simulink model "BESS_grid_test"  (Simulink 8.1)
settings: Solver=ode1  StartTime=0.0  StopTime=inf  FixedStep=Ts  MaxStep=1e-3  RelTol=1e-3
PostLoadFcn:
  | NREL_Mode=3; BANSHEE_init; init_EssTest;
InitFcn:
  | NREL_Mode=3; BANSHEE_init; init_EssTest;
values from neighbouring files (symbols this model uses):
  DER_REL = xlsread('DER_relay.xlsx')    [relay_settings_init.m]
  Ts = 100E-6    (= 0.0001)    [BANSHEE_init.m]    (also in Ghost_init.m)
undefined symbols (not defined in the file or in its folder): CBID, Stim
libraries: simulink x31, breaker_lib x3, rtlab x2, transformer_lib x2, artemis x1, cables_lib x1, BESS_lib x1, relay_modbus_lib x1, rtio_generic_modbus x1, rtio_opalrt_ml605ex1 x1, TestSeq_slave_lib x1, controllable_grid_lib x1
settings Model: ARTEMISmethode_block_infos=$$__separator__$$BESS_grid_test/ARTEMIS Guide$$__separator__$$  Creator=RE25624  LastModifiedBy=pkoralew  BufferReuse=off
settings SolverCC: ZeroCrossAlgorithm=Adaptive
settings DataIOCC: ExternalInput=getinputstruct(op_snapshot1)  InitialState=getstatestruct(op_snapshot1)  LimitDataPoints=off  MaxDataPoints=90060  SignalLoggingSaveFormat=Dataset  SaveOutput=off  SignalLogging=off  DSMLogging=off  SaveTime=off  OutputSaveName=result
settings OptimizationCC: BlockReduction=off  OptimizeBlockIOStorage=off  BufferReuse=off  ExpressionFolding=off  LocalBlockOutputs=off
settings DebuggingCC: MaxConsecutiveZCsMsg=warning  IgnoredZcDiagnostic=none  SolverPrmCheckMsg=none  MultiTaskRateTransMsg=warning  ParameterPrecisionLossMsg=none  FcnCallInpInsideContextMsg=EnableAllAsWarning  FrameProcessingCompatibilityMsg=error  ModelReferenceExtraNoncontSigs=warning
settings ModelReferenceCC: UpdateModelReferenceTargets=IfOutOfDate
settings SFSimCC: SFSimEcho=off
settings GRTTargetCC: CodeReplacementLibrary=C89/C90 (ANSI)

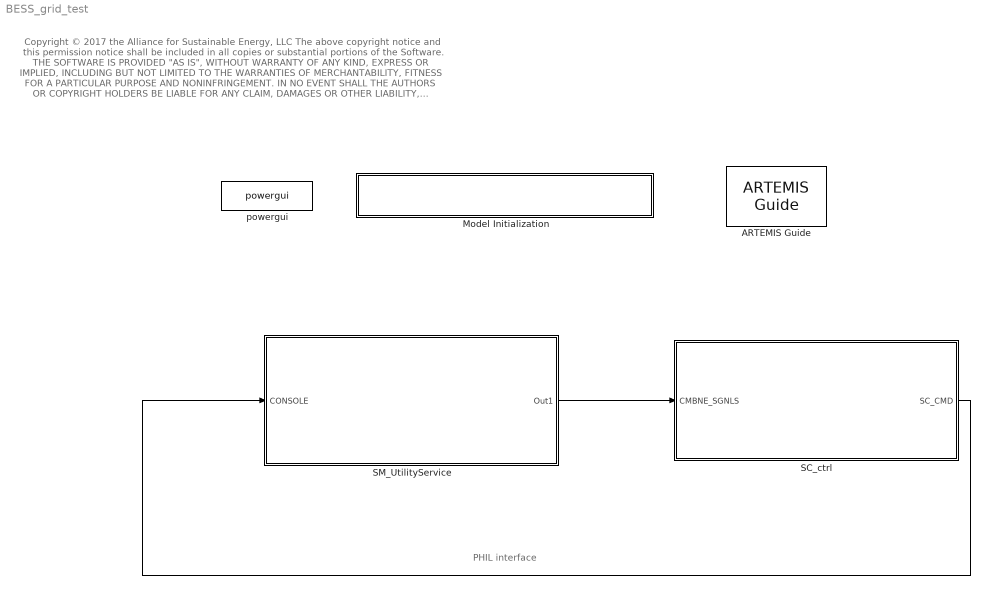
== system BESS_grid_test ==
  note: PHIL interface
  note: Copyright © 2017 the Alliance for Sustainable Energy, LLC
      |
      | The above copyright notice and this permission notice shall be included in all copies or substantial portions of the Software.
      |
      | THE SOFTWARE IS PROVIDED "AS IS", WITHOUT WARRANTY OF ANY KIND, EXPRESS OR IMPLIED, INCLUDING
      | BUT NOT LIMITED TO THE WARRANTIES OF MERCHANTABILITY, FITNESS FOR A PARTICULAR PURPOSE AND
      | NONINFRINGEMENT. IN NO EVENT SHALL THE AUTHORS OR COPYRIGHT HOLDERS BE LIABLE FOR ANY CLAIM,
      |  DAMAGES OR OTHER LIABILITY, WHETHER IN AN ACTION OF CONTRACT, TORT OR OTHERWISE, ARISING FROM,
      | OUT OF OR IN CONNECTION WITH THE SOFTWARE OR THE USE OR OTHER DEALINGS IN THE SOFTWARE
  ARTEMIS Guide : artemis/ARTEMIS/ARTEMIS Guide  Tag=FTSSmethode_opal_4hx0r99  Description=5.0_z1  lock=on  Ts=Ts  opt=art5  dyna=off  nb_perm=4  RT_fullcomp=off  ssn=on  ssn_itvc=off  ssn_ivic=off  ssn_ext=off  ssn_solver=Art5 with Backward Euler nodal interface  ssn_impulse=off  ssn_quasimpulse=off  ssn_impulse_loop=5  paraExtinctionThy=off  Thy_Impulse=on  dtc=Off  dtc_opt=normal  ao=on  simtype=off  ct_mac=off  lin_mov=off  lsp=[0.001 2]  spike_skip=Disabled  dtc_extra=1  dtc_sws=normal  dtc_pied=0.5  SPSRulesBlock=SPSRules  tre=on  ctmm=off  LF=off  dpl_type=ARTEMiS DPL  rlc_type=off  custom_type=off  para=on  ssn_ImpulseLoopBlockedStateUpdate=5  ssn_mov_iter_number=5  ssn_switch_iter_number=5  ssn_nib_type_verify=on
  Model Initialization : Subsystem  AncestorBlock=artemis/Tools /Misc/Model Initialization  mask(Model Functions){InitFcnX=NREL_Mode=3; BANSHEE_init; init_EssTest;, prel=off, posl=on, inif=on, strf=off}
      mask prompts: InitFcnX "Initialisation"; prel "Preload Function"; posl "PostLoad Function"; inif "InitFcn"; strf "StartFcn"
      mask init:
      | currentBlock = gcb;
      | root = bdroot(currentBlock);
      | 
      | if ~strcmp(get_param(root,'BlockDiagramType'),'library')
      |     if prel==1
      |         set_param(root, 'PreLoadFcn', InitFcnX);
      |     else
      |         set_param(root, 'PreLoadFcn', '');
      |     end
      |     if inif==1
      |         set_param(root, 'InitFcn', InitFcnX);
      |     else
      |         set_param(root, 'InitFcn', '');
      |     end
      |     if strf==1
      |         set_param(root, 'StartFcn', InitFcnX);
      |     else
      |         set_param(root, 'StartFcn', '');
      |     end
      |     if posl==1
      |         set_param(root, 'PostLoadFcn', InitFcnX);
      |     else
      |         set_param(root, 'PostLoadFcn', '');
      |     end
      | end
      | 
      | pos = get_param(currentBlock, 'Position');
      | width = pos(3) - pos(1); height = pos(4) - pos(2);
      | txt = [ upper(root) '\n' '- InitFcn. . . . . '  get_param(root, 'InitFcn') ];
      settings: CopyFcn=set_param(gcb,'LinkStatus','inactive')
      mask Display: text(5, height*0.5, txt, 'horizontalAlignment', 'left', 'verticalAlignment', 'middle') ;
  SC_ctrl : Subsystem
  SM_UtilityService : Subsystem
  powergui : powerlib/powergui  Priority=2  SimulationMode=Discrete  SolverType=Tustin  SampleTime=Ts  frequency=60  SPID=off  DisableSnubberDevices=off  DisableRonSwitches=off  DisableVfSwitches=off  SwTol=0  Interpol=off  DisplayEquations=off  frequencyindice=0  Pbase=100e6  ErrMax=1e-4  Iterations=50  UnitsV=kV  UnitsW=MW  FunctionMessages=off  echomessages=off  HookPort=off  EnableUseOfTLC=off  x0status=blocks  RestoreLinks=warning  ResistiveCurrentMeasurement=off  Frange=logspace(0,3,50)  Ylog=off  Xlog=off  ShowGrid=off  save=off  variable=ZData  structure=0  ZoomFFT=on  StartTime=0.0  cycles=2  DisplayStyle=off  fundamental=60  FreqAxis=off  MaxFrequency=1000  frequencyindicesteady=1  RmsSteady=1  display=off  Ts=0  methode=off
  wires:
  SC_ctrl/1(SC_CMD) -> SM_UtilityService/1(CONSOLE)
  SM_UtilityService/1(Out1) -> SC_ctrl/1(CMBNE_SGNLS)

== system BESS_grid_test/Model Initialization ==

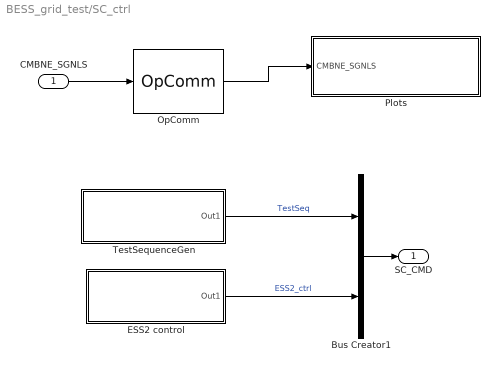
== system BESS_grid_test/SC_ctrl ==
  CMBNE_SGNLS : Inport
  Bus Creator1 : BusCreator  Inputs=2
  ESS2 control : Subsystem
  OpComm : rtlab/OpComm  nbport=1  groupe_acq=1  subsys_rate=0  st=0  Synchronization=on  Interpolation=on  Threshold=1.0  Missed_Data=off  Sim_Time=off  Samples=off  dynSigOut=off  from_console=0  warning_done=off  writeOpCommFile=off  Offset=off
  Plots : Subsystem
  TestSequenceGen : Subsystem
  SC_CMD : Outport
  wires:
  CMBNE_SGNLS/1 -> OpComm/1
  Bus Creator1/1 -> SC_CMD/1
  ESS2 control/1(Out1) -> Bus Creator1/2  "ESS2_ctrl"
  OpComm/1 -> Plots/1(CMBNE_SGNLS)
  TestSequenceGen/1(Out1) -> Bus Creator1/1  "TestSeq"

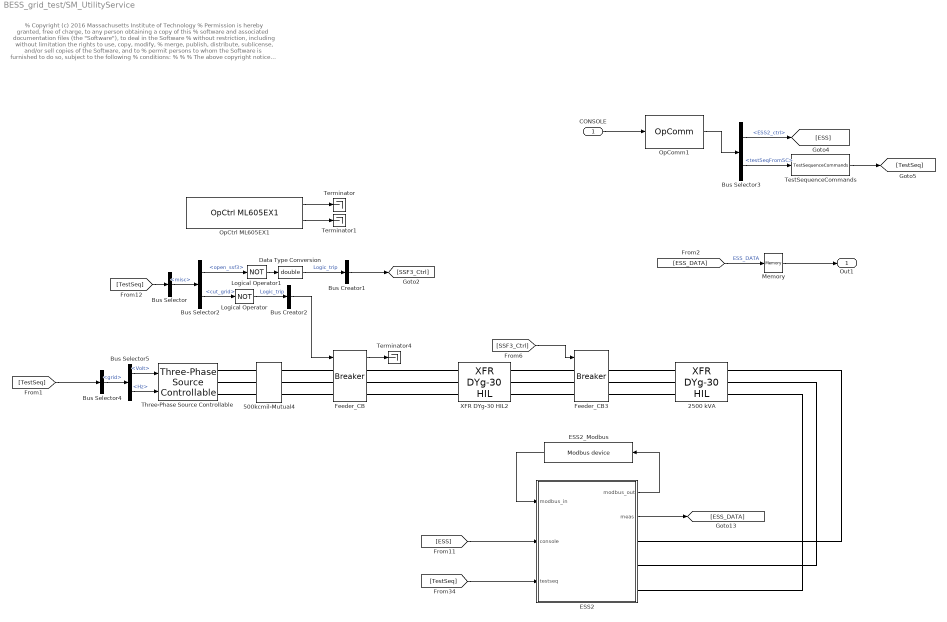
== system BESS_grid_test/SM_UtilityService ==
  note: % Copyright (c) 2016 Massachusetts Institute of Technology
      | % Permission is hereby granted, free of charge, to any person obtaining a copy of this
      | % software and associated documentation files (the "Software"), to deal in the Software
      | % without restriction, including without limitation the rights to use, copy, modify,
      | % merge, publish, distribute, sublicense, and/or sell copies of the Software, and to
      | % permit persons to whom the Software is furnished to do so, subject to the following
      | % conditions:
      | %
      | %
      | % The above copyright notice and this permission notice shall be included in
      | % all copies or substantial portions of the Software.
      | %
      | % THE SOFTWARE IS PROVIDED "AS IS", WITHOUT WARRANTY OF ANY KIND, EXPRESS OR IMPLIED,
      | % INCLUDING BUT NOT LIMITED TO THE WARRANTIES OF MERCHANTABILITY, FITNESS FOR A
      | % PARTICULAR PURPOSE AND NONINFRINGEMENT. IN NO EVENT SHALL THE AUTHORS OR COPYRIGHT
      | % HOLDERS BE LIABLE FOR ANY CLAIM, DAMAGES OR OTHER LIABILITY, WHETHER IN AN ACTION
      | % OF CONTRACT, TORT OR OTHERWISE, ARISING FROM, OUT OF OR IN CONNECTION WITH THE
      | % SOFTWARE OR THE USE OR OTHER DEALINGS IN THE SOFTWARE.
      | %
      | %
      | %%
  CONSOLE : Inport
  2500 kVA : transformer_lib/XFR DYg-30 HIL  Rating=2500  Vp=13800  Vs=480  Z=5.56  XR=5.52
  500kcmil-Mutual4 : cables_lib/500kcmil-Mutual  length=50  par_sets=1  ratio=3
  Bus Creator1 : BusCreator  Inputs=1
  Bus Creator2 : BusCreator  Inputs=1
  Bus Selector : BusSelector  OutputSignals=misc
  Bus Selector2 : BusSelector  OutputSignals=open_ssf3,cut_grid
  Bus Selector3 : BusSelector  OutputSignals=ESS2_ctrl,TestSeq.testSeqFromSC
  Bus Selector4 : BusSelector  OutputSignals=grid
  Bus Selector5 : BusSelector  OutputSignals=Volt,Hz
  Data Type Conversion : DataTypeConversion  OutDataTypeStr=double
  ESS2 : Subsystem
  ESS2_Modbus : rtio_generic_modbus/Modbus device  conf_name=ESS2_modbus.opal  conf_name_mask=ESS2_modbus.xls  sample_time=Ts
  Feeder_CB : breaker_lib/Breaker  Ts=Ts  mech_delay=cb_mech_delay
  Feeder_CB3 : breaker_lib/Breaker  Ts=Ts  mech_delay=cb_mech_delay
  Logical Operator : Logic  Operator=NOT  AllPortsSameDT=off  OutDataTypeStr=boolean
  Logical Operator1 : Logic  Operator=NOT  AllPortsSameDT=off  OutDataTypeStr=boolean
  Memory : Memory
  OpComm1 : rtlab/OpComm  nbport=1  groupe_acq=1  subsys_rate=0  st=0  Synchronization=on  Interpolation=on  Threshold=1.0  Missed_Data=off  Sim_Time=off  Samples=off  dynSigOut=off  from_console=1  warning_done=off  writeOpCommFile=off  Offset=off
  OpCtrl ML605EX1 : rtio_opalrt_ml605ex1/OpCtrl ML605EX1  CtrlName='ML605EX1 Ctrl'  boardid=4  BitstreamFilename=ML605_2-EX-0029-2_2_4_33-32AIO_16DIO16SelectableDIO-10-01.bin  numconfig=-1  mode=Master  externalClock=off  decimRtsi=0  calibIO=off  SampleTime=0  loadinport=-1
  Terminator : Terminator
  Terminator1 : Terminator
  Terminator4 : Terminator
  TestSequenceCommands : TestSeq_slave_lib/TestSequenceCommands
  Three-Phase Source Controllable : controllable_grid_lib/Three-Phase Source Controllable  Ts=Ts  Rg=0.8  Lg=16.58e-3
  XFR DYg-30 HIL2 : transformer_lib/XFR DYg-30 HIL  Rating=50000  Vp=115000  Vs=13800  Z=6  XR=30
  Out1 : Outport
  wires:
  CONSOLE/1 -> OpComm1/1
  OpComm1/1 -> Bus Selector3/1
  Feeder_CB/1 -> Terminator4/1
  [TestSeq] -> Bus Selector/1
  Logical Operator/1 -> Bus Creator2/1  "Logic_trip"
  Bus Creator2/1 -> Feeder_CB/1
  [SSF3_Ctrl] -> Feeder_CB3/1
  OpCtrl ML605EX1/1 -> Terminator/1
  OpCtrl ML605EX1/2 -> Terminator1/1
  Bus Selector/1 -> Bus Selector2/1  "<misc>"
  Bus Selector2/2 -> Logical Operator/1  "<cut_grid>"
  Bus Selector2/1 -> Logical Operator1/1  "<open_ssf3>"
  Logical Operator1/1 -> Data Type Conversion/1
  Bus Creator1/1 -> [SSF3_Ctrl]
  Data Type Conversion/1 -> Bus Creator1/1  "Logic_trip"
  [TestSeq] -> Bus Selector4/1
  Bus Selector4/1 -> Bus Selector5/1  "<grid>"
  Bus Selector5/2 -> Three-Phase Source Controllable/2  "<Hz>"
  Bus Selector5/1 -> Three-Phase Source Controllable/1  "<Volt>"
  [ESS] -> ESS2/2(console)
  ESS2/2(meas) -> [ESS_DATA]
  ESS2/1(modbus_out) -> ESS2_Modbus/1
  ESS2_Modbus/1 -> ESS2/1(modbus_in)
  [TestSeq] -> ESS2/3(testseq)
  [ESS_DATA] -> Memory/1  "ESS_DATA"
  Memory/1 -> Out1/1
  Bus Selector3/1 -> [ESS]  "<ESS2_ctrl>"
  Bus Selector3/2 -> TestSequenceCommands/1  "<testSeqFromSC>"
  TestSequenceCommands/1 -> [TestSeq]
  connections:
  500kcmil-Mutual4/RConn3 -- Feeder_CB/LConn3
  500kcmil-Mutual4/RConn2 -- Feeder_CB/LConn2
  500kcmil-Mutual4/RConn1 -- Feeder_CB/LConn1
  Three-Phase Source Controllable/RConn3 -- 500kcmil-Mutual4/LConn3
  Three-Phase Source Controllable/RConn1 -- 500kcmil-Mutual4/LConn1
  Three-Phase Source Controllable/RConn2 -- 500kcmil-Mutual4/LConn2
  2500 kVA/RConn2 -- ESS2/RConn2
  2500 kVA/RConn1 -- ESS2/RConn1
  2500 kVA/RConn3 -- ESS2/RConn3
  Feeder_CB/RConn1 -- XFR DYg-30 HIL2/LConn1
  Feeder_CB/RConn3 -- XFR DYg-30 HIL2/LConn3
  Feeder_CB/RConn2 -- XFR DYg-30 HIL2/LConn2
  XFR DYg-30 HIL2/RConn2 -- Feeder_CB3/LConn2
  XFR DYg-30 HIL2/RConn3 -- Feeder_CB3/LConn3
  XFR DYg-30 HIL2/RConn1 -- Feeder_CB3/LConn1
  Feeder_CB3/RConn3 -- 2500 kVA/LConn3
  Feeder_CB3/RConn1 -- 2500 kVA/LConn1
  Feeder_CB3/RConn2 -- 2500 kVA/LConn2

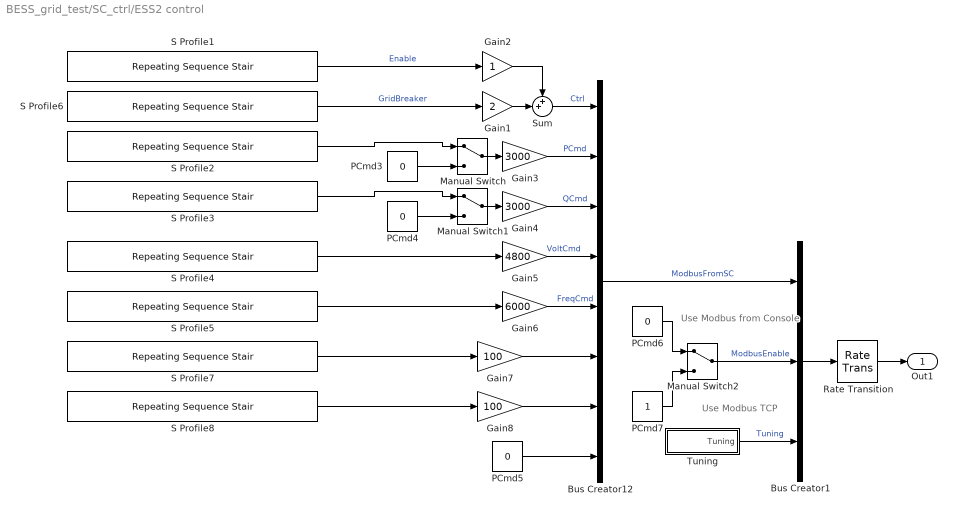
== system BESS_grid_test/SC_ctrl/ESS2 control ==
  note: Use Modbus from
      | Console
  note: Use Modbus TCP
  Bus Creator1 : BusCreator  Inputs=3
  Bus Creator12 : BusCreator  Inputs=8
  Gain1 : Gain  Gain=2
  Gain2 : Gain
  Gain3 : Gain  Gain=3000
  Gain4 : Gain  Gain=3000
  Gain5 : Gain  Gain=4800
  Gain6 : Gain  Gain=6000
  Gain7 : Gain  Gain=100
  Gain8 : Gain  Gain=100
  Manual Switch : ManualSwitch
  Manual Switch1 : ManualSwitch
  Manual Switch2 : ManualSwitch
  PCmd{3..6} (4 alike) : Constant  Value=0
  PCmd7 : Constant
  Rate Transition : RateTransition  Deterministic=off
  S Profile1 : simulink/Sources/Repeating Sequence Stair  OutValues=Stim.ESS.Ena  tsamp=[Stim.Ts Ts]  OutMin=[]  OutMax=[]  OutDataTypeStr=Inherit: Inherit via back propagation  OutDataType=fixdt(0,8)  ConRadixGroup=Best Precision: Vector-wise  OutScaling=2^-12
  S Profile2 : simulink/Sources/Repeating Sequence Stair  OutValues=Stim.ESS.p  tsamp=[Stim.Ts Ts]  OutMin=[]  OutMax=[]  OutDataTypeStr=Inherit: Inherit via back propagation  OutDataType=fixdt(0,8)  ConRadixGroup=Best Precision: Vector-wise  OutScaling=2^-12
  S Profile3 : simulink/Sources/Repeating Sequence Stair  OutValues=Stim.ESS.q  tsamp=[Stim.Ts Ts]  OutMin=[]  OutMax=[]  OutDataTypeStr=Inherit: Inherit via back propagation  OutDataType=fixdt(0,8)  ConRadixGroup=Best Precision: Vector-wise  OutScaling=2^-12
  S Profile4 : simulink/Sources/Repeating Sequence Stair  OutValues=Stim.ESS.v  tsamp=[Stim.Ts Ts]  OutMin=[]  OutMax=[]  OutDataTypeStr=Inherit: Inherit via back propagation  OutDataType=fixdt(0,8)  ConRadixGroup=Best Precision: Vector-wise  OutScaling=2^-12
  S Profile5 : simulink/Sources/Repeating Sequence Stair  OutValues=Stim.ESS.f  tsamp=[Stim.Ts Ts]  OutMin=[]  OutMax=[]  OutDataTypeStr=Inherit: Inherit via back propagation  OutDataType=fixdt(0,8)  ConRadixGroup=Best Precision: Vector-wise  OutScaling=2^-12
  S Profile6 : simulink/Sources/Repeating Sequence Stair  OutValues=Stim.ESS.VFmode  tsamp=[Stim.Ts Ts]  OutMin=[]  OutMax=[]  OutDataTypeStr=Inherit: Inherit via back propagation  OutDataType=fixdt(0,8)  ConRadixGroup=Best Precision: Vector-wise  OutScaling=2^-12
  S Profile7 : simulink/Sources/Repeating Sequence Stair  OutValues=Stim.ESS.D_QV  tsamp=[Stim.Ts Ts]  OutMin=[]  OutMax=[]  OutDataTypeStr=Inherit: Inherit via back propagation  OutDataType=fixdt(0,8)  ConRadixGroup=Best Precision: Vector-wise  OutScaling=2^-12
  S Profile8 : simulink/Sources/Repeating Sequence Stair  OutValues=Stim.ESS.D_PF  tsamp=[Stim.Ts Ts]  OutMin=[]  OutMax=[]  OutDataTypeStr=Inherit: Inherit via back propagation  OutDataType=fixdt(0,8)  ConRadixGroup=Best Precision: Vector-wise  OutScaling=2^-12
  Sum : Sum  Inputs=++|
  Tuning : Subsystem
  Out1 : Outport
  wires:
  S Profile6/1 -> Gain1/1  "GridBreaker"
  S Profile5/1 -> Gain6/1
  Manual Switch/1 -> Gain3/1
  Bus Creator12/1 -> Bus Creator1/1  "ModbusFromSC"
  Manual Switch1/1 -> Gain4/1
  S Profile1/1 -> Gain2/1  "Enable"
  S Profile4/1 -> Gain5/1
  PCmd4/1 -> Manual Switch1/2
  PCmd3/1 -> Manual Switch/2
  S Profile2/1 -> Manual Switch/1
  S Profile3/1 -> Manual Switch1/1
  Gain2/1 -> Sum/1
  Gain1/1 -> Sum/2
  Sum/1 -> Bus Creator12/1  "Ctrl"
  Gain7/1 -> Bus Creator12/6
  Gain8/1 -> Bus Creator12/7
  PCmd5/1 -> Bus Creator12/8
  Bus Creator1/1 -> Rate Transition/1
  Manual Switch2/1 -> Bus Creator1/2  "ModbusEnable"
  PCmd6/1 -> Manual Switch2/1
  PCmd7/1 -> Manual Switch2/2
  Gain3/1 -> Bus Creator12/2  "PCmd"
  Gain4/1 -> Bus Creator12/3  "QCmd"
  Gain5/1 -> Bus Creator12/4  "VoltCmd"
  Gain6/1 -> Bus Creator12/5  "FreqCmd"
  Rate Transition/1 -> Out1/1
  Tuning/1(Tuning) -> Bus Creator1/3  "Tuning"
  S Profile7/1 -> Gain7/1
  S Profile8/1 -> Gain8/1

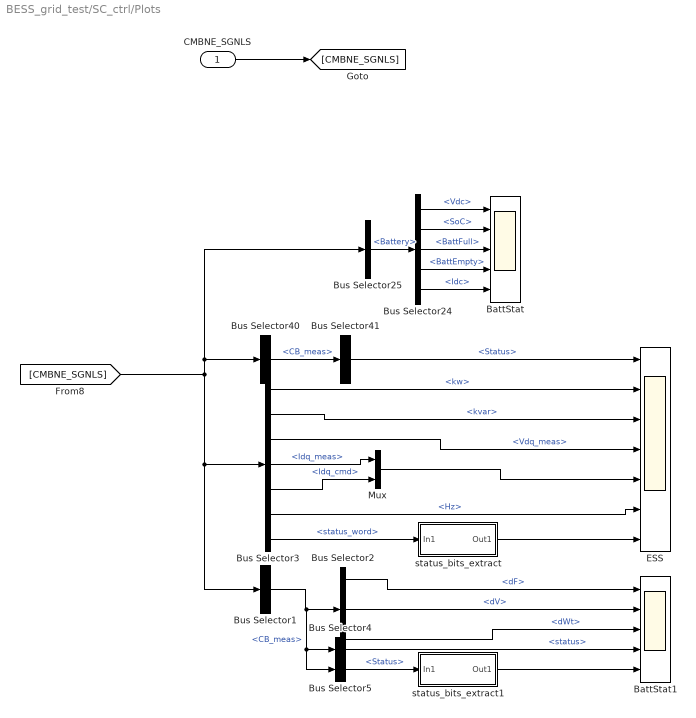
== system BESS_grid_test/SC_ctrl/Plots ==
  CMBNE_SGNLS : Inport
  BattStat : Scope  NumInputPorts=5
      settings: YMin=-1~-1~-1~49.9984~-5  YMax=1~1~1~49.9985~5  SaveName=ScopeData11  Decimation=Stim.Dec
  BattStat1 : Scope  NumInputPorts=5
      settings: YMin=-60~-8~-100~0~0  YMax=30~3~800~17500~11  Decimation=Stim.Dec
  Bus Selector1 : BusSelector  OutputSignals=CB_meas
  Bus Selector2 : BusSelector  OutputSignals=relay_meas.dF,relay_meas.dV,relay_meas.dWt
  Bus Selector24 : BusSelector  OutputSignals=Vdc,SoC,BattFull,BattEmpty,Idc
  Bus Selector25 : BusSelector  OutputSignals=Battery
  Bus Selector3 : BusSelector  OutputSignals=CB_meas.relay_out.m.kw,CB_meas.relay_out.m.kvar,Inverter.Vdq_meas,Inverter.Idq_meas,Inverter.Idq_cmd,CB_meas.relay_out.m.Hz,status_word
  Bus Selector4 : BusSelector  OutputSignals=relay_out.m.status
  Bus Selector40 : BusSelector  OutputSignals=CB_meas
  Bus Selector41 : BusSelector  OutputSignals=cb_meas.Status
  Bus Selector5 : BusSelector  OutputSignals=cb_meas.Status
  ESS : Scope  NumInputPorts=7
      settings: YMin=0~-500~-20~-100~-2000~59.8~0  YMax=1~3000~90~500~6000~60.15~12.5  SaveName=ScopeData13  Decimation=Stim.Dec
  Mux : Mux  Inputs=2
  status_bits_extract : Subsystem
  status_bits_extract1 : Subsystem
  wires:
  CMBNE_SGNLS/1 -> [CMBNE_SGNLS]
  Bus Selector3/4 -> Mux/1  "<Idq_meas>"
  Mux/1 -> ESS/5
  Bus Selector3/3 -> ESS/4  "<Vdq_meas>"
  Bus Selector24/2 -> BattStat/2  "<SoC>"
  Bus Selector24/1 -> BattStat/1  "<Vdc>"
  Bus Selector24/3 -> BattStat/3  "<BattFull>"
  Bus Selector24/4 -> BattStat/4  "<BattEmpty>"
  Bus Selector25/1 -> Bus Selector24/1  "<Battery>"
  Bus Selector3/5 -> Mux/2  "<Idq_cmd>"
  Bus Selector3/6 -> ESS/6  "<Hz>"
  Bus Selector3/1 -> ESS/2  "<kw>"
  Bus Selector3/2 -> ESS/3  "<kvar>"
  Bus Selector41/1 -> ESS/1  "<Status>"
  Bus Selector40/1 -> Bus Selector41/1  "<CB_meas>"
  Bus Selector24/5 -> BattStat/5  "<Idc>"
  status_bits_extract/1(Out1) -> ESS/7
  Bus Selector3/7 -> status_bits_extract/1(In1)  "<status_word>"
  [CMBNE_SGNLS] -> Bus Selector1/1, Bus Selector3/1, Bus Selector25/1, Bus Selector40/1
  Bus Selector1/1 -> Bus Selector5/1, Bus Selector4/1, Bus Selector2/1  "<CB_meas>"
  Bus Selector2/2 -> BattStat1/2  "<dV>"
  Bus Selector2/3 -> BattStat1/3  "<dWt>"
  Bus Selector2/1 -> BattStat1/1  "<dF>"
  Bus Selector4/1 -> BattStat1/4  "<status>"
  Bus Selector5/1 -> status_bits_extract1/1(In1)  "<Status>"
  status_bits_extract1/1(Out1) -> BattStat1/5

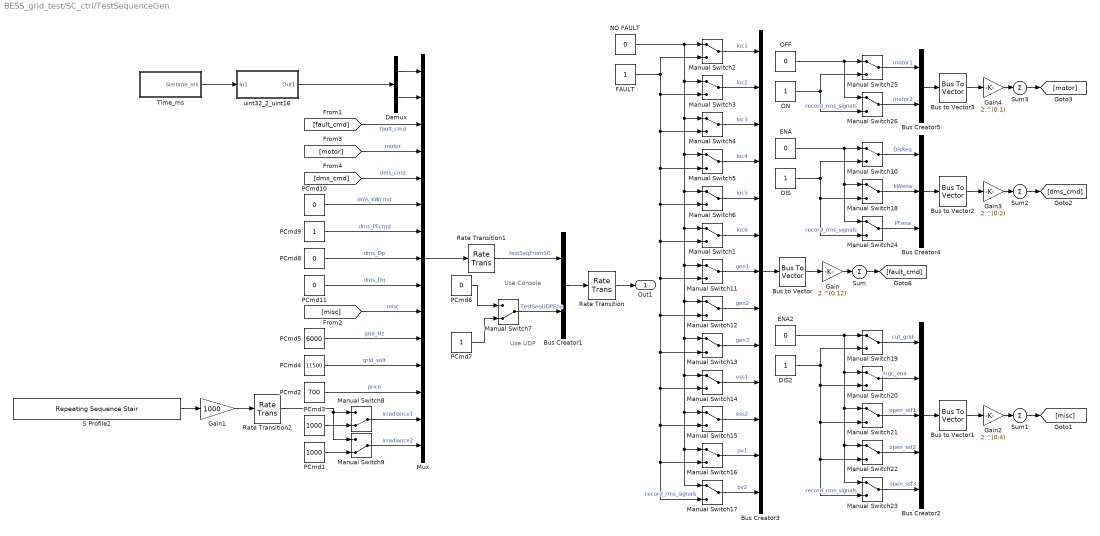
== system BESS_grid_test/SC_ctrl/TestSequenceGen ==
  note: Use Console
  note: Use UDP
  Bus Creator1 : BusCreator  Inputs=2
  Bus Creator2 : BusCreator  Inputs=5
  Bus Creator3 : BusCreator  Inputs=13
  Bus Creator4 : BusCreator  Inputs=3
  Bus Creator5 : BusCreator  Inputs=2
  Bus to Vector{,1..3} (4 alike) : BusToVector
  DIS : Constant
  DIS2 : Constant
  Demux : Demux  Outputs=2
  ENA : Constant  Value=0
  ENA2 : Constant  Value=0
  FAULT : Constant
  Gain : Gain  Gain=2.^(0:12)
  Gain1 : Gain  Gain=1000
  Gain2 : Gain  Gain=2.^(0:4)
  Gain3 : Gain  Gain=2.^(0:2)
  Gain4 : Gain  Gain=2.^(0:1)
  Manual Switch{1..6,10..26} (23 alike) : ManualSwitch
  Manual Switch7 : ManualSwitch  CurrentSetting=0
  Manual Switch8 : ManualSwitch  CurrentSetting=0
  Manual Switch9 : ManualSwitch  CurrentSetting=0
  Mux : Mux  Inputs=15
  NO FAULT : Constant  Value=0
  OFF : Constant  Value=0
  ON : Constant
  PCmd1 : Constant  Value=1000
  PCmd10 : Constant  Value=0
  PCmd11 : Constant  Value=0
  PCmd2 : Constant  Value=700
  PCmd3 : Constant  Value=1000
  PCmd4 : Constant  Value=11500
  PCmd5 : Constant  Value=6000
  PCmd6 : Constant  Value=0  SampleTime=[Stim.Ts Ts]
  PCmd7 : Constant
  PCmd8 : Constant  Value=0
  PCmd9 : Constant
  Rate Transition : RateTransition  Deterministic=off
  Rate Transition1 : RateTransition  Deterministic=off  OutPortSampleTime=1e-2
  Rate Transition2 : RateTransition  Deterministic=off  OutPortSampleTime=1e-2
  S Profile2 : simulink/Sources/Repeating Sequence Stair  OutValues=Stim.PV2.Irradiance  tsamp=[Stim.Ts Ts]  OutMin=[]  OutMax=[]  OutDataTypeStr=Inherit: Inherit via back propagation  OutDataType=fixdt(0,8)  ConRadixGroup=Best Precision: Vector-wise  OutScaling=2^-12
  Sum{,1..3} (4 alike) : Sum  Inputs=+
  Time_ms : Subsystem
  uint32_2_uint16 : Subsystem
      mask Display: disp('uint32_2_uint16');
  Out1 : Outport
  wires:
  Manual Switch4/1 -> Bus Creator3/3  "loc3"
  Manual Switch5/1 -> Bus Creator3/4  "loc4"
  [fault_cmd] -> Mux/3  "fault_cmd"
  Bus Creator3/1 -> Bus to Vector/1
  Manual Switch2/1 -> Bus Creator3/1  "loc1"
  Manual Switch6/1 -> Bus Creator3/5  "loc5"
  Manual Switch3/1 -> Bus Creator3/2  "loc2"
  Manual Switch1/1 -> Bus Creator3/6  "loc6"
  Manual Switch13/1 -> Bus Creator3/9  "gen3"
  Manual Switch14/1 -> Bus Creator3/10  "ess1"
  Manual Switch11/1 -> Bus Creator3/7  "gen1"
  Manual Switch15/1 -> Bus Creator3/11  "ess2"
  Manual Switch12/1 -> Bus Creator3/8  "gen2"
  FAULT/1 -> Manual Switch2/2, Manual Switch1/2, Manual Switch12/2, Manual Switch13/2, Manual Switch14/2, Manual Switch17/2, Manual Switch16/2, Manual Switch15/2, Manual Switch11/2, Manual Switch6/2, Manual Switch5/2, Manual Switch4/2, Manual Switch3/2  "record_rms_signals"
  NO FAULT/1 -> Manual Switch12/1, Manual Switch13/1, Manual Switch14/1, Manual Switch15/1, Manual Switch17/1, Manual Switch16/1, Manual Switch11/1, Manual Switch1/1, Manual Switch6/1, Manual Switch5/1, Manual Switch4/1, Manual Switch3/1, Manual Switch2/1
  Manual Switch16/1 -> Bus Creator3/12  "pv1"
  Manual Switch17/1 -> Bus Creator3/13  "pv2"
  Bus to Vector/1 -> Gain/1
  Gain/1 -> Sum/1
  Sum/1 -> [fault_cmd]
  Mux/1 -> Rate Transition1/1
  Bus Creator1/1 -> Rate Transition/1
  Manual Switch7/1 -> Bus Creator1/2  "TestSeqUDPEna"
  PCmd6/1 -> Manual Switch7/1
  PCmd7/1 -> Manual Switch7/2
  Rate Transition/1 -> Out1/1
  PCmd3/1 -> Manual Switch8/2
  Manual Switch9/1 -> Mux/15  "irradiance2"
  PCmd1/1 -> Manual Switch9/2
  Manual Switch8/1 -> Mux/14  "irradiance1"
  PCmd2/1 -> Mux/13  "price"
  Gain1/1 -> Rate Transition2/1
  Time_ms/1(Simtime_ms) -> uint32_2_uint16/1(In1)
  Demux/1 -> Mux/1
  Demux/2 -> Mux/2
  PCmd4/1 -> Mux/12  "grid_volt"
  PCmd5/1 -> Mux/11  "grid_Hz"
  [misc] -> Mux/10  "misc"
  [motor] -> Mux/4  "motor"
  [dms_cmd] -> Mux/5  "dms_cmd"
  PCmd8/1 -> Mux/8  "dms_Dp"
  PCmd9/1 -> Mux/7  "dms_PFcmd"
  PCmd10/1 -> Mux/6  "dms_kWcmd"
  PCmd11/1 -> Mux/9  "dms_Dq"
  Manual Switch21/1 -> Bus Creator2/3  "open_ssf1"
  Manual Switch22/1 -> Bus Creator2/4  "open_ssf2"
  Bus Creator2/1 -> Bus to Vector1/1
  Manual Switch19/1 -> Bus Creator2/1  "cut_grid"
  Manual Switch23/1 -> Bus Creator2/5  "open_ssf3"
  Manual Switch20/1 -> Bus Creator2/2  "mgc_ena"
  DIS2/1 -> Manual Switch20/2, Manual Switch21/2, Manual Switch22/2, Manual Switch23/2, Manual Switch19/2  "record_rms_signals"
  ENA2/1 -> Manual Switch19/1, Manual Switch20/1, Manual Switch21/1, Manual Switch22/1, Manual Switch23/1
  Bus to Vector1/1 -> Gain2/1
  Gain2/1 -> Sum1/1
  Sum1/1 -> [misc]
  Manual Switch24/1 -> Bus Creator4/3  "PFena"
  Bus Creator4/1 -> Bus to Vector2/1
  Manual Switch10/1 -> Bus Creator4/1  "DisReq"
  Manual Switch18/1 -> Bus Creator4/2  "kWena"
  DIS/1 -> Manual Switch10/2, Manual Switch24/2, Manual Switch18/2  "record_rms_signals"
  ENA/1 -> Manual Switch24/1, Manual Switch18/1, Manual Switch10/1
  Bus to Vector2/1 -> Gain3/1
  Gain3/1 -> Sum2/1
  Sum2/1 -> [dms_cmd]
  Bus Creator5/1 -> Bus to Vector3/1
  Manual Switch25/1 -> Bus Creator5/1  "motor1"
  Manual Switch26/1 -> Bus Creator5/2  "motor2"
  ON/1 -> Manual Switch26/2, Manual Switch25/2  "record_rms_signals"
  OFF/1 -> Manual Switch25/1, Manual Switch26/1
  Bus to Vector3/1 -> Gain4/1
  Gain4/1 -> Sum3/1
  Sum3/1 -> [motor]
  S Profile2/1 -> Gain1/1
  uint32_2_uint16/1(Out1) -> Demux/1
  Rate Transition1/1 -> Bus Creator1/1  "testSeqFromSC"
  Rate Transition2/1 -> Manual Switch9/1, Manual Switch8/1

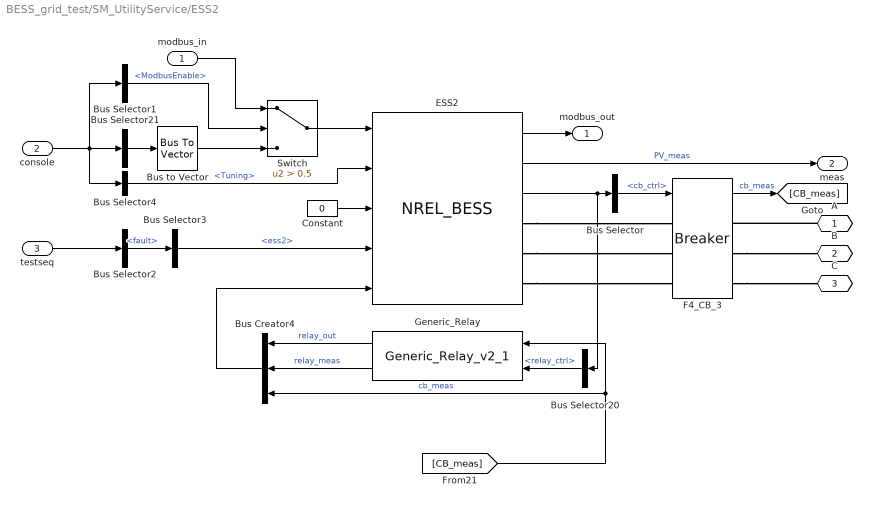
== system BESS_grid_test/SM_UtilityService/ESS2 ==
  modbus_in : Inport
  console : Inport  Port=2
  testseq : Inport  Port=3
  Bus Creator4 : BusCreator  Inputs=3
  Bus Selector : BusSelector  OutputSignals=cb_ctrl
  Bus Selector1 : BusSelector  OutputSignals=ModbusEnable
  Bus Selector2 : BusSelector  OutputSignals=fault
  Bus Selector20 : BusSelector  OutputSignals=relay_ctrl
  Bus Selector21 : BusSelector  OutputSignals=ModbusFromSC.Ctrl,ModbusFromSC.PCmd,ModbusFromSC.QCmd,ModbusFromSC.VoltCmd,ModbusFromSC.FreqCmd,ModbusFromSC.signal6,ModbusFromSC.signal7,ModbusFromSC.signal8  OutputAsBus=on
  Bus Selector3 : BusSelector  OutputSignals=ess2
  Bus Selector4 : BusSelector  OutputSignals=Tuning
  Bus to Vector : BusToVector
  Constant : Constant  Value=0
  ESS2 : BESS_lib/NREL_BESS  InvType=ESS Inverter  Sn=3000  Vn=480  b_Vdc_nom=1000  b_kWh=600  b_esr=0.1  r_I_max=3  Tc=Ts  MbusPrecInc=off  ExtTuningEna=on
  F4_CB_3 : breaker_lib/Breaker  Ts=Ts  mech_delay=cb_mech_delay
  Generic_Relay : relay_modbus_lib/Generic_Relay_v2_1  Ts=Ts  relay_settings=[DER_REL(CBID.ESS1,:)]
  Switch : Switch  Criteria=u2 > Threshold  Threshold=0.5
  A : PMIOPort  Port=1  Side=Right
  B : PMIOPort  Port=2  Side=Right
  C : PMIOPort  Port=3  Side=Right
  modbus_out : Outport
  meas : Outport  Port=2
  wires:
  Bus Creator4/1 -> ESS2/5
  Generic_Relay/2 -> Bus Creator4/2  "relay_meas"
  ESS2/2 -> meas/1  "PV_meas"
  Generic_Relay/1 -> Bus Creator4/1  "relay_out"
  Bus Selector20/1 -> Generic_Relay/2  "<relay_ctrl>"
  console/1 -> Bus Selector4/1, Bus Selector1/1, Bus Selector21/1
  Bus Selector1/1 -> Switch/2  "<ModbusEnable>"
  ESS2/1 -> modbus_out/1
  modbus_in/1 -> Switch/1
  Bus Selector21/1 -> Bus to Vector/1
  Switch/1 -> ESS2/1
  ESS2/3 -> Bus Selector20/1, Bus Selector/1
  Bus to Vector/1 -> Switch/3
  Constant/1 -> ESS2/3
  testseq/1 -> Bus Selector2/1
  Bus Selector2/1 -> Bus Selector3/1  "<fault>"
  Bus Selector3/1 -> ESS2/4  "<ess2>"
  [CB_meas] -> Generic_Relay/1, Bus Creator4/3  "cb_meas"
  F4_CB_3/1 -> [CB_meas]  "cb_meas"
  Bus Selector/1 -> F4_CB_3/1  "<cb_ctrl>"
  Bus Selector4/1 -> ESS2/2  "<Tuning>"
  connections:
  F4_CB_3/RConn2 -- B/RConn1
  ESS2/RConn2 -- F4_CB_3/LConn2
  ESS2/RConn3 -- F4_CB_3/LConn3
  ESS2/RConn1 -- F4_CB_3/LConn1
  A/RConn1 -- F4_CB_3/RConn1
  F4_CB_3/RConn3 -- C/RConn1

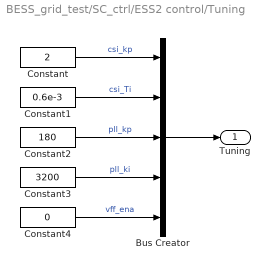
== system BESS_grid_test/SC_ctrl/ESS2 control/Tuning ==
  Bus Creator : BusCreator  Inputs=5
  Constant : Constant  Value=2  SampleTime=[Stim.Ts Ts]
  Constant1 : Constant  Value=0.6e-3  SampleTime=[Stim.Ts Ts]
  Constant2 : Constant  Value=180  SampleTime=[Stim.Ts Ts]
  Constant3 : Constant  Value=3200  SampleTime=[Stim.Ts Ts]
  Constant4 : Constant  Value=0  SampleTime=[Stim.Ts Ts]
  Tuning : Outport
  wires:
  Bus Creator/1 -> Tuning/1
  Constant/1 -> Bus Creator/1  "csi_kp"
  Constant1/1 -> Bus Creator/2  "csi_Ti"
  Constant2/1 -> Bus Creator/3  "pll_kp"
  Constant3/1 -> Bus Creator/4  "pll_ki"
  Constant4/1 -> Bus Creator/5  "vff_ena"

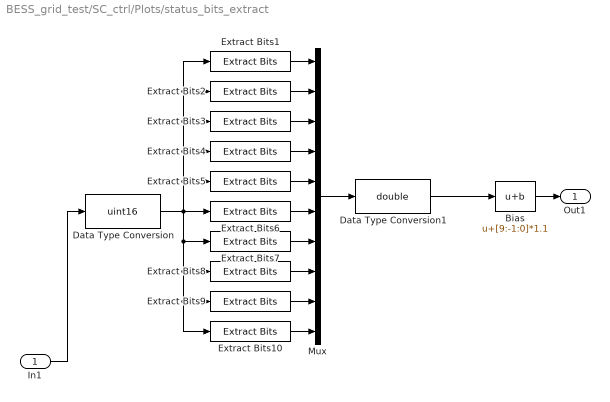
== system BESS_grid_test/SC_ctrl/Plots/status_bits_extract ==
  In1 : Inport
  Bias : Bias  Bias=[9:-1:0]*1.1
  Data Type Conversion : DataTypeConversion  OutDataTypeStr=uint16
  Data Type Conversion1 : DataTypeConversion  OutDataTypeStr=double
  Extract Bits1 : simulink/Logic and Bit Operations/Extract Bits  bitsToExtract=Range of bits  numBits=8  bitIdxRange=0  outScalingMode=Treat bit field as an integer
  Extract Bits10 : simulink/Logic and Bit Operations/Extract Bits  bitsToExtract=Range of bits  numBits=8  bitIdxRange=9  outScalingMode=Treat bit field as an integer
  Extract Bits2 : simulink/Logic and Bit Operations/Extract Bits  bitsToExtract=Range of bits  numBits=8  bitIdxRange=1  outScalingMode=Treat bit field as an integer
  Extract Bits3 : simulink/Logic and Bit Operations/Extract Bits  bitsToExtract=Range of bits  numBits=8  bitIdxRange=2  outScalingMode=Treat bit field as an integer
  Extract Bits4 : simulink/Logic and Bit Operations/Extract Bits  bitsToExtract=Range of bits  numBits=8  bitIdxRange=3  outScalingMode=Treat bit field as an integer
  Extract Bits5 : simulink/Logic and Bit Operations/Extract Bits  bitsToExtract=Range of bits  numBits=8  bitIdxRange=4  outScalingMode=Treat bit field as an integer
  Extract Bits6 : simulink/Logic and Bit Operations/Extract Bits  bitsToExtract=Range of bits  numBits=8  bitIdxRange=5  outScalingMode=Treat bit field as an integer
  Extract Bits7 : simulink/Logic and Bit Operations/Extract Bits  bitsToExtract=Range of bits  numBits=8  bitIdxRange=6  outScalingMode=Treat bit field as an integer
  Extract Bits8 : simulink/Logic and Bit Operations/Extract Bits  bitsToExtract=Range of bits  numBits=8  bitIdxRange=7  outScalingMode=Treat bit field as an integer
  Extract Bits9 : simulink/Logic and Bit Operations/Extract Bits  bitsToExtract=Range of bits  numBits=8  bitIdxRange=8  outScalingMode=Treat bit field as an integer
  Mux : Mux  Inputs=10
  Out1 : Outport
  wires:
  Bias/1 -> Out1/1
  Extract Bits5/1 -> Mux/5
  In1/1 -> Data Type Conversion/1
  Extract Bits2/1 -> Mux/2
  Data Type Conversion/1 -> Extract Bits1/1, Extract Bits2/1, Extract Bits3/1, Extract Bits4/1, Extract Bits5/1, Extract Bits8/1, Extract Bits10/1, Extract Bits9/1, Extract Bits7/1, Extract Bits6/1
  Mux/1 -> Data Type Conversion1/1
  Extract Bits1/1 -> Mux/1
  Data Type Conversion1/1 -> Bias/1
  Extract Bits10/1 -> Mux/10
  Extract Bits8/1 -> Mux/8
  Extract Bits9/1 -> Mux/9
  Extract Bits3/1 -> Mux/3
  Extract Bits4/1 -> Mux/4
  Extract Bits7/1 -> Mux/7
  Extract Bits6/1 -> Mux/6

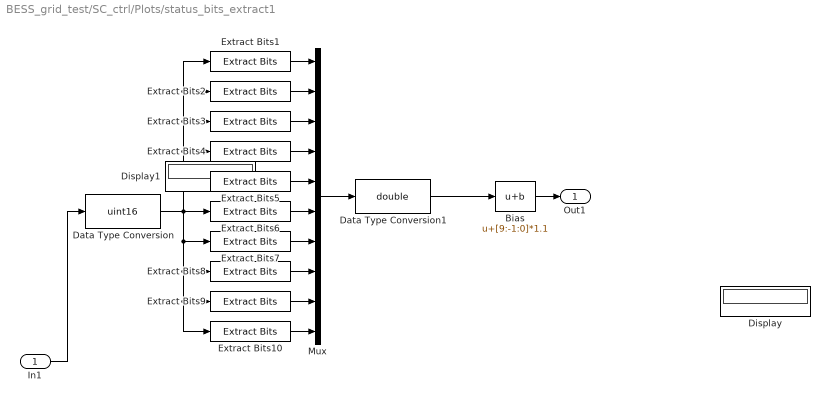
== system BESS_grid_test/SC_ctrl/Plots/status_bits_extract1 ==
  In1 : Inport
  Bias : Bias  Bias=[9:-1:0]*1.1
  Data Type Conversion : DataTypeConversion  OutDataTypeStr=uint16
  Data Type Conversion1 : DataTypeConversion  OutDataTypeStr=double
  Display : Display
  Display1 : Display
  Extract Bits1 : simulink/Logic and Bit Operations/Extract Bits  bitsToExtract=Range of bits  numBits=8  bitIdxRange=0  outScalingMode=Treat bit field as an integer
  Extract Bits10 : simulink/Logic and Bit Operations/Extract Bits  bitsToExtract=Range of bits  numBits=8  bitIdxRange=9  outScalingMode=Treat bit field as an integer
  Extract Bits2 : simulink/Logic and Bit Operations/Extract Bits  bitsToExtract=Range of bits  numBits=8  bitIdxRange=1  outScalingMode=Treat bit field as an integer
  Extract Bits3 : simulink/Logic and Bit Operations/Extract Bits  bitsToExtract=Range of bits  numBits=8  bitIdxRange=2  outScalingMode=Treat bit field as an integer
  Extract Bits4 : simulink/Logic and Bit Operations/Extract Bits  bitsToExtract=Range of bits  numBits=8  bitIdxRange=3  outScalingMode=Treat bit field as an integer
  Extract Bits5 : simulink/Logic and Bit Operations/Extract Bits  bitsToExtract=Range of bits  numBits=8  bitIdxRange=4  outScalingMode=Treat bit field as an integer
  Extract Bits6 : simulink/Logic and Bit Operations/Extract Bits  bitsToExtract=Range of bits  numBits=8  bitIdxRange=5  outScalingMode=Treat bit field as an integer
  Extract Bits7 : simulink/Logic and Bit Operations/Extract Bits  bitsToExtract=Range of bits  numBits=8  bitIdxRange=6  outScalingMode=Treat bit field as an integer
  Extract Bits8 : simulink/Logic and Bit Operations/Extract Bits  bitsToExtract=Range of bits  numBits=8  bitIdxRange=7  outScalingMode=Treat bit field as an integer
  Extract Bits9 : simulink/Logic and Bit Operations/Extract Bits  bitsToExtract=Range of bits  numBits=8  bitIdxRange=8  outScalingMode=Treat bit field as an integer
  Mux : Mux  Inputs=10
  Out1 : Outport
  wires:
  Extract Bits6/1 -> Mux/6
  Extract Bits7/1 -> Mux/7
  Extract Bits4/1 -> Mux/4
  Extract Bits3/1 -> Mux/3
  Extract Bits9/1 -> Mux/9
  Extract Bits8/1 -> Mux/8
  Extract Bits10/1 -> Mux/10
  Data Type Conversion1/1 -> Bias/1
  Extract Bits1/1 -> Mux/1
  Mux/1 -> Data Type Conversion1/1
  Data Type Conversion/1 -> Extract Bits6/1, Extract Bits7/1, Extract Bits9/1, Extract Bits10/1, Extract Bits8/1, Extract Bits5/1, Extract Bits4/1, Extract Bits3/1, Extract Bits2/1, Extract Bits1/1
  Extract Bits2/1 -> Mux/2
  In1/1 -> Data Type Conversion/1
  Extract Bits5/1 -> Mux/5
  Bias/1 -> Out1/1

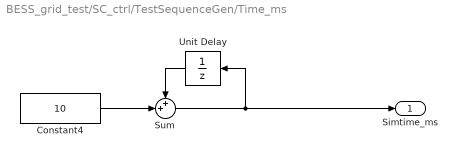
== system BESS_grid_test/SC_ctrl/TestSequenceGen/Time_ms ==
  Constant4 : Constant  Value=10
  Sum : Sum  Inputs=++|
  Unit Delay : UnitDelay  SampleTime=1e-2
  Simtime_ms : Outport
  wires:
  Unit Delay/1 -> Sum/1
  Constant4/1 -> Sum/2
  Sum/1 -> Unit Delay/1, Simtime_ms/1

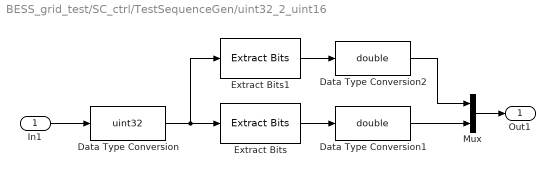
== system BESS_grid_test/SC_ctrl/TestSequenceGen/uint32_2_uint16 ==
  In1 : Inport
  Data Type Conversion : DataTypeConversion  OutDataTypeStr=uint32
  Data Type Conversion1 : DataTypeConversion  OutDataTypeStr=double
  Data Type Conversion2 : DataTypeConversion  OutDataTypeStr=double
  Extract Bits : simulink/Logic and Bit Operations/Extract Bits  bitsToExtract=Upper half  numBits=8  bitIdxRange=[0 7]  outScalingMode=Treat bit field as an integer
  Extract Bits1 : simulink/Logic and Bit Operations/Extract Bits  bitsToExtract=Lower half  numBits=8  bitIdxRange=[0 7]  outScalingMode=Preserve fixed-point scaling
  Mux : Mux  Inputs=2
  Out1 : Outport
  wires:
  Extract Bits1/1 -> Data Type Conversion2/1
  Data Type Conversion1/1 -> Mux/2
  Data Type Conversion2/1 -> Mux/1
  Data Type Conversion/1 -> Extract Bits/1, Extract Bits1/1
  In1/1 -> Data Type Conversion/1
  Extract Bits/1 -> Data Type Conversion1/1
  Mux/1 -> Out1/1
